simulink model "lqg_linearsys"  (R2019b)
settings: Solver=VariableStepAuto  StartTime=0.0  StopTime=60  RelTol=1e-3
values from neighbouring files (symbols this model uses):
  K_theta = tf(lqg_ss)    [rocket_controllerdesign.m]
  sys = ss(A,B,C,D)    [controller_design.m]    (also in main_yp_fminunc.m; rocket_controllerdesign.m; rocket_controllerdesign_z.m; rocket_model.m)
settings Model: Creator=bia  LastModifiedBy=bia

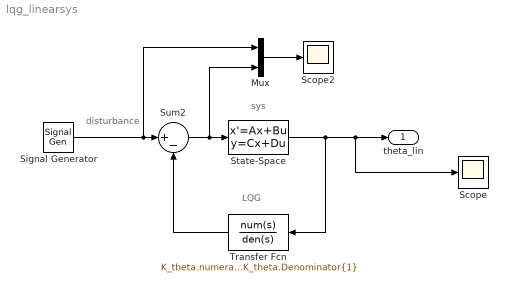
== system lqg_linearsys ==
  note: LQG
  note: sys
  note: disturbance
  Mux : Mux  Inputs=2
  Scope : Scope
  Scope2 : Scope
  Signal Generator : SignalGenerator  WaveForm=square  Amplitude=1e-6  Units=rad/sec
  State-Space : StateSpace  A=sys.A  B=sys.B  C=sys.C  D=sys.D  InitialCondition=0
  Sum2 : Sum  Inputs=|+-
  Transfer Fcn : TransferFcn  Numerator=K_theta.numerator{1}  Denominator=K_theta.Denominator{1}
  theta_lin : Outport
  wires:
  State-Space/1 -> Transfer Fcn/1, Scope/1, theta_lin/1
  Signal Generator/1 -> Mux/1, Sum2/1
  Sum2/1 -> Mux/2, State-Space/1
  Transfer Fcn/1 -> Sum2/2
  Mux/1 -> Scope2/1
